simulink model "three_pole"  (R2025a)
settings: Solver=VariableStepAuto  StartTime=0.0  StopTime=10  RelTol=1e-3
undefined symbols (not defined in the file): alpha, beta, Ki, Kp, leff, wn
settings Model: Creator=julianshah  LastModifiedBy=julianshah

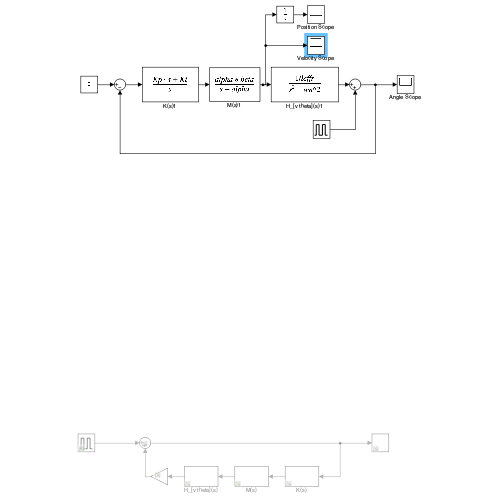
[thumbnail: Simulink's stored preview of the top-level diagram]
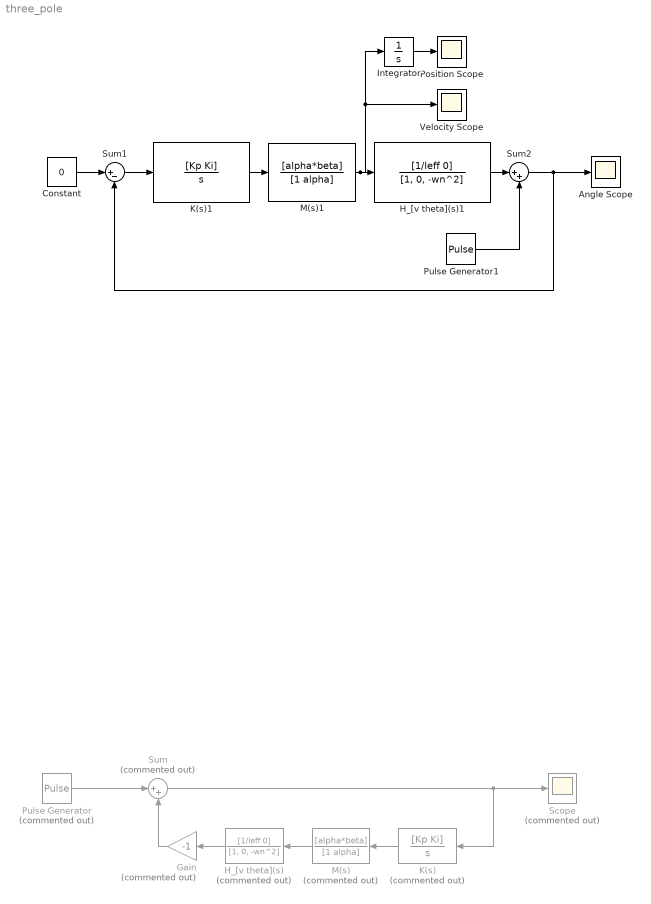
== system three_pole ==
  Angle Scope : Scope
      settings: ActiveDisplayYMinimum=-14.671967690347316  ActiveDisplayYMaximum=16.659154055795813
  Constant : Constant  Value=0
  Gain : Gain  Commented=on  Gain=-1
  H_[v theta](s) : TransferFcn  Commented=on  Numerator=[1/leff 0]  Denominator=[1, 0, -wn^2]
  H_[v theta](s)1 : TransferFcn  Numerator=[1/leff 0]  Denominator=[1, 0, -wn^2]
  Integrator : Integrator
  K(s) : TransferFcn  Commented=on  Numerator=[Kp Ki]  Denominator=[1, 0]
  K(s)1 : TransferFcn  Numerator=[Kp Ki]  Denominator=[1, 0]
  M(s) : TransferFcn  Commented=on  Numerator=[alpha*beta]  Denominator=[1 alpha]
  M(s)1 : TransferFcn  Numerator=[alpha*beta]  Denominator=[1 alpha]
  Position Scope : Scope
      settings: ActiveDisplayYMinimum=-65.260573740284983  ActiveDisplayYMaximum=190.93468961900868  DataLoggingVariableName=ScopeData3
  Pulse Generator : DiscretePulseGenerator  Commented=on  PulseType=Time based  Amplitude=100000000  Period=50
  Pulse Generator1 : DiscretePulseGenerator  PulseType=Time based  PulseWidth=5
  Scope : Scope  Commented=on
      settings: ActiveDisplayYMinimum=4.5536739794630995E+9  ActiveDisplayYMaximum=5.0189998204162264E+9
  Sum : Sum  Commented=on  Inputs=|++
  Sum1 : Sum  Inputs=|+-
  Sum2 : Sum  Inputs=|++
  Velocity Scope : Scope
      settings: ActiveDisplayYMinimum=-10.923785344159537  ActiveDisplayYMaximum=28.739021550726218  DataLoggingVariableName=ScopeData2
  wires:
  Pulse Generator/1 -> Sum/1
  K(s)/1 -> M(s)/1
  M(s)/1 -> H_[v theta](s)/1
  H_[v theta](s)/1 -> Gain/1
  Gain/1 -> Sum/2
  Sum/1 -> K(s)/1, Scope/1
  M(s)1/1 -> Integrator/1, Velocity Scope/1, H_[v theta](s)1/1
  K(s)1/1 -> M(s)1/1
  Sum1/1 -> K(s)1/1
  Pulse Generator1/1 -> Sum2/2
  Sum2/1 -> Sum1/2, Angle Scope/1
  Constant/1 -> Sum1/1
  H_[v theta](s)1/1 -> Sum2/1
  Integrator/1 -> Position Scope/1
